simulink model "sys4_LA"  (R2023a)
settings: Solver=ode15s  StartTime=0.0  StopTime=10  MaxStep=1E-3  RelTol=1e-3
settings Model: LastModifiedBy=edgar
settings DataIOCC: ReturnWorkspaceOutputs=off  TimeSaveName=t
settings DebuggingCC: AlgebraicLoopMsg=none  ArtificialAlgebraicLoopMsg=none  MaxConsecutiveZCsMsg=none  ModelReferenceExtraNoncontSigs=none  OperatingPointInterfaceChecksumMismatchMsg=none
settings RTWCC: GPUComputeCapability=5.0

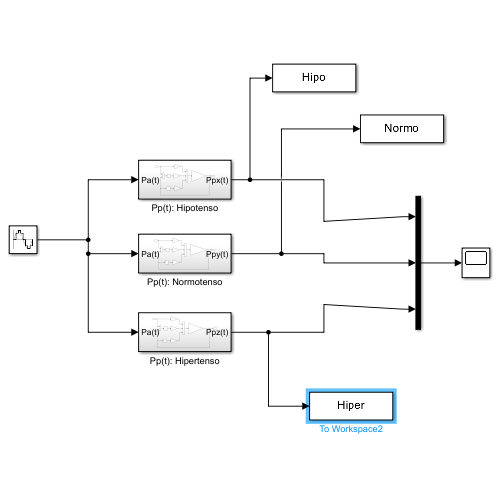
[thumbnail: Simulink's stored preview of the top-level diagram]
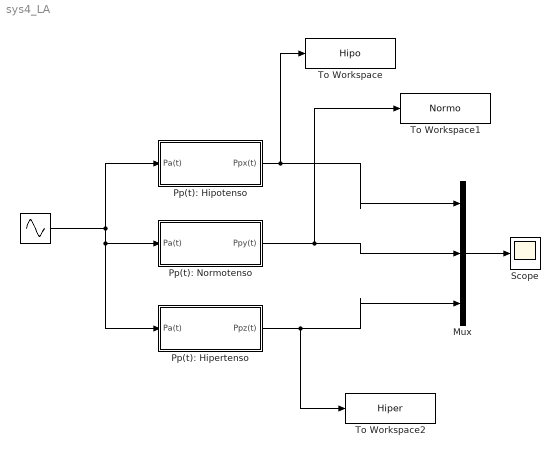
== system sys4_LA ==
  " " : Sin  Bias=0.8  Frequency=2*pi*(95/60)  SampleTime=0.001
  Mux : Mux  Inputs=3
  Pp(t): Hipertenso : Subsystem
  Pp(t): Hipotenso : Subsystem
  Pp(t): Normotenso : Subsystem
  Scope : Scope
  To Workspace : ToWorkspace  VariableName=Hipo  SampleTime=-1
  To Workspace1 : ToWorkspace  VariableName=Normo  SampleTime=-1
  To Workspace2 : ToWorkspace  VariableName=Hiper  SampleTime=-1
  wires:
  Mux/1 -> Scope/1
  Pp(t): Normotenso/1(Ppy(t)) -> To Workspace1/1, Mux/2
  Pp(t): Hipotenso/1(Ppx(t)) -> To Workspace/1, Mux/1
  Pp(t): Hipertenso/1(Ppz(t)) -> To Workspace2/1, Mux/3
  " "/1 -> Pp(t): Hipertenso/1(Pa(t)), Pp(t): Normotenso/1(Pa(t)), Pp(t): Hipotenso/1(Pa(t))

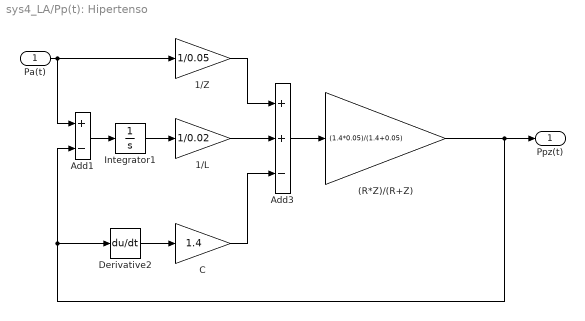
== system sys4_LA/Pp(t): Hipertenso ==
  Pa(t) : Inport
  (R*Z)/(R+Z) : Gain  Gain=(1.4*0.05)/(1.4+0.05)
  1/L : Gain  Gain=1/0.02
  1/Z : Gain  Gain=1/0.05
  Add1 : Sum  Inputs=+-
  Add3 : Sum  Inputs=++-
  C : Gain  Gain=1.4
  Derivative2 : Derivative
  Integrator1 : Integrator
  Ppz(t) : Outport
  wires:
  Add3/1 -> (R*Z)/(R+Z)/1
  Add1/1 -> Integrator1/1
  Integrator1/1 -> 1/L/1
  1/L/1 -> Add3/2
  Pa(t)/1 -> 1/Z/1, Add1/1
  1/Z/1 -> Add3/1
  (R*Z)/(R+Z)/1 -> Ppz(t)/1, Add1/2, Derivative2/1
  Derivative2/1 -> C/1
  C/1 -> Add3/3

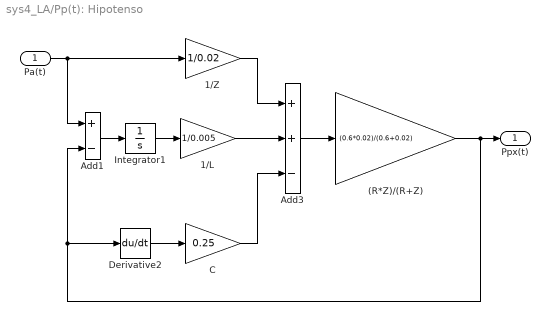
== system sys4_LA/Pp(t): Hipotenso ==
  Pa(t) : Inport
  (R*Z)/(R+Z) : Gain  Gain=(0.6*0.02)/(0.6+0.02)
  1/L : Gain  Gain=1/0.005
  1/Z : Gain  Gain=1/0.02
  Add1 : Sum  Inputs=+-
  Add3 : Sum  Inputs=++-
  C : Gain  Gain=0.25
  Derivative2 : Derivative
  Integrator1 : Integrator
  Ppx(t) : Outport
  wires:
  Add3/1 -> (R*Z)/(R+Z)/1
  Add1/1 -> Integrator1/1
  Integrator1/1 -> 1/L/1
  1/L/1 -> Add3/2
  Pa(t)/1 -> 1/Z/1, Add1/1
  1/Z/1 -> Add3/1
  (R*Z)/(R+Z)/1 -> Ppx(t)/1, Add1/2, Derivative2/1
  Derivative2/1 -> C/1
  C/1 -> Add3/3

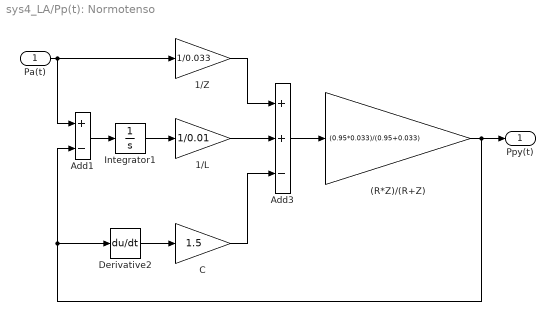
== system sys4_LA/Pp(t): Normotenso ==
  Pa(t) : Inport
  (R*Z)/(R+Z) : Gain  Gain=(0.95*0.033)/(0.95+0.033)
  1/L : Gain  Gain=1/0.01
  1/Z : Gain  Gain=1/0.033
  Add1 : Sum  Inputs=+-
  Add3 : Sum  Inputs=++-
  C : Gain  Gain=1.5
  Derivative2 : Derivative
  Integrator1 : Integrator
  Ppy(t) : Outport
  wires:
  Add3/1 -> (R*Z)/(R+Z)/1
  Add1/1 -> Integrator1/1
  Integrator1/1 -> 1/L/1
  1/L/1 -> Add3/2
  Pa(t)/1 -> 1/Z/1, Add1/1
  1/Z/1 -> Add3/1
  (R*Z)/(R+Z)/1 -> Add1/2, Derivative2/1, Ppy(t)/1
  Derivative2/1 -> C/1
  C/1 -> Add3/3
